simulink model "SPGF_FSK_0000_R2020b"  (R2020b)
settings: Solver=ode4  StartTime=0.0  StopTime=1.4  FixedStep=50e-6/50  RelTol=1e-3  EnableMultiTasking=on
undefined symbols (not defined in the file): D11, Delta
libraries: powerlib x2546, powerlib_meascontrol x183, simulink x24
(part 20 of 34)

== system SPGF_FSK_0000_R2020b/W31/DPL ==
  Ccs2/1 : powerlib/Elements/Series RLC Branch  LConnTagsString=__new0  RConnTagsString=__new0  BranchType=R  Resistance=-Rg_matrix(3,4)*2  Inductance=1e-3  SetiL0=off  InitialCurrent=0  Capacitance=Rg_matrix(3,4)*2  Setx0=off  InitialVoltage=0  Measurements=None
  Ccs2/3 : powerlib/Elements/Series RLC Branch  LConnTagsString=__new0  RConnTagsString=__new0  BranchType=R  Resistance=-Rg_matrix(3,4)*2  Inductance=1e-3  SetiL0=off  InitialCurrent=0  Capacitance=Rg_matrix(3,4)*2  Setx0=off  InitialVoltage=0  Measurements=None
  Ccs3/1 : powerlib/Elements/Series RLC Branch  LConnTagsString=__new0  RConnTagsString=__new0  BranchType=R  Resistance=-Rg_matrix(5,6)*2  Inductance=1e-3  SetiL0=off  InitialCurrent=0  Capacitance=-C_matrix(5,6)/2  Setx0=off  InitialVoltage=0  Measurements=None
  Ccs3/3 : powerlib/Elements/Series RLC Branch  LConnTagsString=__new0  RConnTagsString=__new0  BranchType=R  Resistance=-Rg_matrix(5,6)*2  Inductance=1e-3  SetiL0=off  InitialCurrent=0  Capacitance=-C_matrix(5,6)/2  Setx0=off  InitialVoltage=0  Measurements=None
  DPL : powerlib/Elements/Distributed Parameters Line  Phases=6  Length=LineLength  Frequency=Frequency  Resistance=R_matrix  Inductance=L_matrix  Capacitance=C_matrix  x1=[-3.15e-05 -1.16357054266887 0 -12.5014827360038 0 0 -9092.8182742179;-3.1e-05 -1.16390866949271 0 -12.505151651317 0 0 -9092.02733285201;-3.05e-05 -1.16424676759825 0 -12.5088202580778 0 0 -9091.23616714935;-3e-05 -1.16458483697715 0 -12.5124885561959 0 0 -9090.44477712942;-2.95e-05 -1.16492287762107 0 -12.5161565455808 0 0 -9089.65316281176;-2.9e-05 -1.16526088952168 0 -12.5198242261418 0 0 -9088.86132421589;-2.85e-05 -1.16559887267062 0 -12.5234915977886 0 0 -9088.06926136137;-2.8e-05 -1.16593682705957 0 -12.5271586604306 0 0 -9087.27697426772;-2.75e-05 -1.16627475268017 0 -12.5308254139773 0 0 -9086.4844629545;-2.7e-05 -1.1666126495241 0 -12.5344918583383 0 0 -9085.69172744126;-2.65e-05 -1.16695051758302 0 -12.5381579934231 0 0 -9084.89876774757;-2.6e-05 -1.16728835684859 0 -12.5418238191413 0 0 -9084.10558389299;-2.55e-05 -1.16762616731247 0 -12.5454893354024 0 0 -9083.31217589708;-2.5e-05 -1.16796394896633 0 -12.5491545421159 0 0 -9082.51854377943;-2.45e-05 -1.16830170180183 0 -12.5528194391915 0 0 -9081.72468755962;-2.4e-05 -1.16863942581065 0 -12.5564840265387 0 0 -9080.93060725724;-2.35e-05 -1.16897712098445 0 -12.560148304067 0 0 -9080.13630289187;-2.3e-05 -1.16931478731489 0 -12.5638122716861 0 0 -9079.34177448312;-2.25e-05 -1.16965242479364 0 -12.5674759293056 0 0 -9078.54702205059;-2.2e-05 -1.16999003341238 0 -12.571139276835 0 0 -9077.75204561389;-2.15e-05 -1.17032761316277 0 -12.574802314184 0 0 -9076.95684519264;-2.1e-05 -1.17066516403648 0 -12.5784650412621 0 0 -9076.16142080646;-2.05e-05 -1.17100268602519 0 -12.5821274579791 0 0 -9075.36577247497;-2e-05 -1.17134017912057 0 -12.5857895642446 0 0 -9074.56990021781;-1.95e-05 -1.17167764331428 0 -12.5894513599681 0 0 -9073.77380405461;-1.9e-05 -1.17201507859801 0 -12.5931128450594 0 0 -9072.97748400501;-1.85e-05 -1.17235248496343 0 -12.5967740194281 0 0 -9072.18094008867;-1.8e-05 -1.17268986240221 0 -12.6004348829838 0 0 -9071.38417232524;-1.75e-05 -1.17302721090602 0 -12.6040954356363 0 0 -9070.58718073438;-1.7e-05 -1.17336453046655 0 -12.6077556772951 0 0 -9069.78996533574;-1.65e-05 -1.17370182107547 0 -12.6114156078701 0 0 -9068.99252614901;-1.6e-05 -1.17403908272446 0 -12.6150752272709 0 0 -9068.19486319386;-1.55e-05 -1.17437631540519 0 -12.6187345354071 0 0 -9067.39697648997;-1.5e-05 -1.17471351910935 0 -12.6223935321886 0 0 -9066.59886605703;-1.45e-05 -1.17505069382862 0 -12.626052217525 0 0 -9065.80053191473;-1.4e-05 -1.17538783955467 0 -12.629710591326 0 0 -9065.00197408277;-1.35e-05 -1.17572495627919 0 -12.6333686535014 0 0 -9064.20319258085;-1.3e-05 -1.17606204399386 0 -12.637026403961 0 0 -9063.40418742868;-1.25e-05 -1.17639910269037 0 -12.6406838426144 0 0 -9062.60495864597;-1.2e-05 -1.17673613236039 0 -12.6443409693714 0 0 -9061.80550625245;-1.15e-05 -1.1770731329956 0 -12.6479977841419 0 0 -9061.00583026785;-1.1e-05 -1.17741010458771 0 -12.6516542868355 0 0 -9060.20593071188;-1.05e-05 -1.17774704712838 0 -12.655310477362 0 0 -9059.4058076043;-1e-05 -1.17808396060931 0 -12.6589663556313 0 0 -9058.60546096484;-9.5e-06 -1.17842084502218 0 -12.6626219215531 0 0 -9057.80489081324;-9e-06 -1.17875770035868 0 -12.6662771750372 0 0 -9057.00409716928;-8.5e-06 -1.17909452661051 0 -12.6699321159935 0 0 -9056.20308005269;-8e-06 -1.17943132376934 0 -12.6735867443317 0 0 -9055.40183948325;-7.5e-06 -1.17976809182687 0 -12.6772410599617 0 0 -9054.60037548072;-7e-06 -1.18010483077479 0 -12.6808950627934 0 0 -9053.79868806488;-6.5e-06 -1.18044154060479 0 -12.6845487527364 0 0 -9052.99677725552;-6e-06 -1.18077822130856 0 -12.6882021297008 0 0 -9052.19464307242;-5.5e-06 -1.1811148728778 5103.15019671596 -12.6918551935964 -2795.65081043936 4961.78174708621 -9051.39228553536;-5e-06 -1.1814514953042 5104.5723005975 -12.6955079443329 -2796.42987939011 4961.34178923313 -9050.58970466416;-4.5e-06 -1.18178808857945 5105.99427852876 -12.6991603818204 -2797.20887934172 4960.90170896385 -9049.7869004786;-4e-06 -1.18212465269524 5107.41613047466 -12.7028125059687 ...(+845 chars)]  x2=[-3.15e-05 -1.16269751442728 0 -12.461505127574 0 0 -9158.28571557594;-3.1e-05 -1.16304211630014 0 -12.4652625773679 0 0 -9157.49238310332;-3.05e-05 -1.16338668947608 0 -12.4690197195937 0 0 -9156.69882467864;-3e-05 -1.1637312339466 0 -12.4727765541588 0 0 -9155.90504032147;-2.95e-05 -1.16407574970321 0 -12.4765330809705 0 0 -9155.11103005139;-2.9e-05 -1.1644202367374 0 -12.480289299936 0 0 -9154.31679388801;-2.85e-05 -1.16476469504067 0 -12.4840452109628 0 0 -9153.52233185092;-2.8e-05 -1.16510912460452 0 -12.4878008139581 0 0 -9152.72764395971;-2.75e-05 -1.16545352542046 0 -12.4915561088292 0 0 -9151.932730234;-2.7e-05 -1.16579789747999 0 -12.4953110954836 0 0 -9151.1375906934;-2.65e-05 -1.1661422407746 0 -12.4990657738285 0 0 -9150.34222535754;-2.6e-05 -1.16648655529581 0 -12.5028201437714 0 0 -9149.54663424603;-2.55e-05 -1.16683084103512 0 -12.5065742052195 0 0 -9148.7508173785;-2.5e-05 -1.16717509798403 0 -12.5103279580803 0 0 -9147.9547747746;-2.45e-05 -1.16751932613405 0 -12.5140814022611 0 0 -9147.15850645397;-2.4e-05 -1.16786352547669 0 -12.5178345376693 0 0 -9146.36201243624;-2.35e-05 -1.16820769600344 0 -12.5215873642123 0 0 -9145.56529274108;-2.3e-05 -1.16855183770583 0 -12.5253398817976 0 0 -9144.76834738813;-2.25e-05 -1.16889595057536 0 -12.5290920903324 0 0 -9143.97117639708;-2.2e-05 -1.16924003460353 0 -12.5328439897244 0 0 -9143.17377978758;-2.15e-05 -1.16958408978187 0 -12.5365955798807 0 0 -9142.37615757931;-2.1e-05 -1.16992811610187 0 -12.540346860709 0 0 -9141.57830979194;-2.05e-05 -1.17027211355506 0 -12.5440978321167 0 0 -9140.78023644518;-2e-05 -1.17061608213293 0 -12.5478484940111 0 0 -9139.9819375587;-1.95e-05 -1.17096002182702 0 -12.5515988462998 0 0 -9139.18341315222;-1.9e-05 -1.17130393262882 0 -12.5553488888902 0 0 -9138.38466324541;-1.85e-05 -1.17164781452986 0 -12.5590986216898 0 0 -9137.58568785801;-1.8e-05 -1.17199166752164 0 -12.562848044606 0 0 -9136.78648700971;-1.75e-05 -1.17233549159569 0 -12.5665971575464 0 0 -9135.98706072025;-1.7e-05 -1.17267928674353 0 -12.5703459604184 0 0 -9135.18740900934;-1.65e-05 -1.17302305295666 0 -12.5740944531296 0 0 -9134.38753189672;-1.6e-05 -1.1733667902266 0 -12.5778426355874 0 0 -9133.58742940212;-1.55e-05 -1.17371049854489 0 -12.5815905076994 0 0 -9132.78710154528;-1.5e-05 -1.17405417790302 0 -12.5853380693731 0 0 -9131.98654834595;-1.45e-05 -1.17439782829253 0 -12.5890853205161 0 0 -9131.18576982389;-1.4e-05 -1.17474144970494 0 -12.5928322610358 0 0 -9130.38476599885;-1.35e-05 -1.17508504213176 0 -12.5965788908398 0 0 -9129.5835368906;-1.3e-05 -1.17542860556452 0 -12.6003252098357 0 0 -9128.7820825189;-1.25e-05 -1.17577213999474 0 -12.6040712179311 0 0 -9127.98040290353;-1.2e-05 -1.17611564541395 0 -12.6078169150334 0 0 -9127.17849806428;-1.15e-05 -1.17645912181367 0 -12.6115623010503 0 0 -9126.37636802092;-1.1e-05 -1.17680256918542 0 -12.6153073758894 0 0 -9125.57401279325;-1.05e-05 -1.17714598752073 0 -12.6190521394583 0 0 -9124.77143240107;-1e-05 -1.17748937681113 0 -12.6227965916646 0 0 -9123.96862686418;-9.5e-06 -1.17783273704815 0 -12.6265407324158 0 0 -9123.16559620239;-9e-06 -1.1781760682233 0 -12.6302845616196 0 0 -9122.3623404355;-8.5e-06 -1.17851937032813 0 -12.6340280791837 0 0 -9121.55885958335;-8e-06 -1.17886264335416 0 -12.6377712850155 0 0 -9120.75515366576;-7.5e-06 -1.17920588729292 0 -12.6415141790229 0 0 -9119.95122270256;-7e-06 -1.17954910213593 0 -12.6452567611135 0 0 -9119.14706671358;-6.5e-06 -1.17989228787475 0 -12.6489990311948 0 0 -9118.34268571866;-6e-06 -1.18023544450088 0 -12.6527409891746 0 0 -9117.53807973766;-5.5e-06 -1.18057857200588 5127.76906785034 -12.6564826349605 -2809.1377281476 4997.60028069833 -9116.73324879042;-5e-06 -1.18092167038126 5129.20187253766 -12.6602239684602 -2809.92265930412 4997.15896609033 -9115.9281928968;-4.5e-06 -1.18126473961857 5130.63455066699 -12.6639649895814 -2810.70752112858 4996.71752818238 -9115.12291207668;-4e-06 -1.18160777970934 5132.06710220299 -12.6677056982318 -2811.49231360161 ...(+828 chars)]  x3=[-3.15e-05 0.0167006451886816 0 -0.592002992330624 0 0 -460.167467556111;-3.1e-05 0.0166975880195327 0 -0.592580585093426 0 0 -460.166571304681;-3.05e-05 0.0166945304383873 0 -0.593158163234887 0 0 -460.165663699096;-3e-05 0.0166914724453209 0 -0.593735726740758 0 0 -460.164744739379;-2.95e-05 0.0166884140404089 0 -0.594313275596787 0 0 -460.163814425552;-2.9e-05 0.0166853552237268 0 -0.594890809788724 0 0 -460.162872757637;-2.85e-05 0.0166822959953501 0 -0.595468329302319 0 0 -460.161919735659;-2.8e-05 0.0166792363553542 0 -0.596045834123321 0 0 -460.160955359641;-2.75e-05 0.0166761763038147 0 -0.596623324237482 0 0 -460.159979629606;-2.7e-05 0.0166731158408069 0 -0.597200799630553 0 0 -460.158992545579;-2.65e-05 0.0166700549664066 0 -0.597778260288284 0 0 -460.157994107584;-2.6e-05 0.0166669936806891 0 -0.598355706196428 0 0 -460.156984315645;-2.55e-05 0.0166639319837301 0 -0.598933137340737 0 0 -460.155963169788;-2.5e-05 0.016660869875605 0 -0.599510553706963 0 0 -460.154930670038;-2.45e-05 0.0166578073563894 0 -0.600087955280859 0 0 -460.15388681642;-2.4e-05 0.0166547444261589 0 -0.600665342048179 0 0 -460.15283160896;-2.35e-05 0.0166516810849891 0 -0.601242713994675 0 0 -460.151765047684;-2.3e-05 0.0166486173329555 0 -0.601820071106101 0 0 -460.150687132618;-2.25e-05 0.0166455531701337 0 -0.602397413368213 0 0 -460.149597863789;-2.2e-05 0.0166424885965993 0 -0.602974740766764 0 0 -460.148497241224;-2.15e-05 0.0166394236124281 0 -0.603552053287511 0 0 -460.147385264949;-2.1e-05 0.0166363582176955 0 -0.604129350916207 0 0 -460.146261934994;-2.05e-05 0.0166332924124772 0 -0.604706633638609 0 0 -460.145127251384;-2e-05 0.0166302261968489 0 -0.605283901440472 0 0 -460.143981214148;-1.95e-05 0.0166271595708861 0 -0.605861154307554 0 0 -460.142823823315;-1.9e-05 0.0166240925346647 0 -0.606438392225612 0 0 -460.141655078912;-1.85e-05 0.0166210250882603 0 -0.607015615180401 0 0 -460.14047498097;-1.8e-05 0.0166179572317484 0 -0.607592823157681 0 0 -460.139283529516;-1.75e-05 0.0166148889652049 0 -0.608170016143209 0 0 -460.138080724581;-1.7e-05 0.0166118202887055 0 -0.608747194122744 0 0 -460.136866566193;-1.65e-05 0.0166087512023258 0 -0.609324357082043 0 0 -460.135641054384;-1.6e-05 0.0166056817061417 0 -0.609901505006866 0 0 -460.134404189182;-1.55e-05 0.0166026118002287 0 -0.610478637882974 0 0 -460.133155970619;-1.5e-05 0.0165995414846627 0 -0.611055755696124 0 0 -460.131896398726;-1.45e-05 0.0165964707595195 0 -0.611632858432078 0 0 -460.130625473533;-1.4e-05 0.0165933996248748 0 -0.612209946076596 0 0 -460.129343195073;-1.35e-05 0.0165903280808043 0 -0.612787018615439 0 0 -460.128049563375;-1.3e-05 0.0165872561273839 0 -0.613364076034369 0 0 -460.126744578474;-1.25e-05 0.0165841837646893 0 -0.613941118319147 0 0 -460.125428240399;-1.2e-05 0.0165811109927965 0 -0.614518145455535 0 0 -460.124100549185;-1.15e-05 0.0165780378117811 0 -0.615095157429295 0 0 -460.122761504864;-1.1e-05 0.016574964221719 0 -0.615672154226191 0 0 -460.121411107469;-1.05e-05 0.0165718902226861 0 -0.616249135831985 0 0 -460.120049357033;-1e-05 0.0165688158147581 0 -0.616826102232442 0 0 -460.11867625359;-9.5e-06 0.0165657409980111 0 -0.617403053413324 0 0 -460.117291797174;-9e-06 0.0165626657725207 0 -0.617979989360397 0 0 -460.115895987819;-8.5e-06 0.016559590138363 0 -0.618556910059424 0 0 -460.114488825558;-8e-06 0.0165565140956137 0 -0.619133815496172 0 0 -460.113070310429;-7.5e-06 0.0165534376443489 0 -0.619710705656405 0 0 -460.111640442464;-7e-06 0.0165503607846443 0 -0.62028758052589 0 0 -460.110199221699;-6.5e-06 0.016547283516576 0 -0.620864440090392 0 0 -460.10874664817;-6e-06 0.0165442058402198 0 -0.621441284335677 0 0 -460.107282721913;-5.5e-06 0.0165411277556516 -10.2033229098497 -0.622018113247514 -286.489948414025 588.173233513661 -460.105807442964;-5e-06 0.0165380492629475 -10.1348731635547 -0.622594926811669 -286.578402750177 588.127601544154 -460.10432081136;-4.5e-06 0.0165349703621835 -10.0664231671918 -0.62317172501391 ...(+981 chars)]  x4=[-3.15e-05 -0.0306851840034263 0 -1.23273715720339 0 0 174.215498589481;-3.1e-05 -0.0306862799089198 0 -1.23270367838231 0 0 174.239382593604;-3.05e-05 -0.0306873750572597 0 -1.23267016914548 0 0 174.263262298543;-3e-05 -0.0306884694484189 0 -1.23263662949374 0 0 174.287137703709;-2.95e-05 -0.0306895630823705 0 -1.23260305942791 0 0 174.311008808512;-2.9e-05 -0.0306906559590875 0 -1.23256945894881 0 0 174.334875612363;-2.85e-05 -0.0306917480785429 0 -1.23253582805729 0 0 174.358738114674;-2.8e-05 -0.0306928394407098 0 -1.23250216675416 0 0 174.382596314855;-2.75e-05 -0.0306939300455612 0 -1.23246847504026 0 0 174.406450212318;-2.7e-05 -0.0306950198930703 0 -1.23243475291642 0 0 174.430299806474;-2.65e-05 -0.0306961089832101 0 -1.23240100038347 0 0 174.454145096735;-2.6e-05 -0.0306971973159538 0 -1.23236721744224 0 0 174.477986082513;-2.55e-05 -0.0306982848912745 0 -1.23233340409358 0 0 174.501822763219;-2.5e-05 -0.0306993717091454 0 -1.2322995603383 0 0 174.525655138265;-2.45e-05 -0.0307004577695396 0 -1.23226568617725 0 0 174.549483207063;-2.4e-05 -0.0307015430724304 0 -1.23223178161127 0 0 174.573306969025;-2.35e-05 -0.0307026276177911 0 -1.23219784664118 0 0 174.597126423564;-2.3e-05 -0.0307037114055947 0 -1.23216388126783 0 0 174.620941570091;-2.25e-05 -0.0307047944358146 0 -1.23212988549206 0 0 174.644752408019;-2.2e-05 -0.0307058767084241 0 -1.2320958593147 0 0 174.668558936761;-2.15e-05 -0.0307069582233964 0 -1.23206180273659 0 0 174.692361155729;-2.1e-05 -0.030708038980705 0 -1.23202771575858 0 0 174.716159064335;-2.05e-05 -0.030709118980323 0 -1.2319935983815 0 0 174.739952661993;-2e-05 -0.0307101982222239 0 -1.23195945060619 0 0 174.763741948116;-1.95e-05 -0.030711276706381 0 -1.23192527243351 0 0 174.787526922116;-1.9e-05 -0.0307123544327678 0 -1.23189106386429 0 0 174.811307583406;-1.85e-05 -0.0307134314013576 0 -1.23185682489938 0 0 174.835083931401;-1.8e-05 -0.0307145076121238 0 -1.23182255553961 0 0 174.858855965513;-1.75e-05 -0.03071558306504 0 -1.23178825578585 0 0 174.882623685155;-1.7e-05 -0.0307166577600795 0 -1.23175392563892 0 0 174.906387089742;-1.65e-05 -0.0307177316972158 0 -1.23171956509969 0 0 174.930146178687;-1.6e-05 -0.0307188048764226 0 -1.23168517416899 0 0 174.953900951403;-1.55e-05 -0.0307198772976731 0 -1.23165075284768 0 0 174.977651407305;-1.5e-05 -0.0307209489609411 0 -1.23161630113661 0 0 175.001397545806;-1.45e-05 -0.0307220198662001 0 -1.23158181903662 0 0 175.025139366321;-1.4e-05 -0.0307230900134236 0 -1.23154730654857 0 0 175.048876868263;-1.35e-05 -0.0307241594025853 0 -1.23151276367331 0 0 175.072610051048;-1.3e-05 -0.0307252280336587 0 -1.23147819041169 0 0 175.09633891409;-1.25e-05 -0.0307262959066175 0 -1.23144358676456 0 0 175.120063456802;-1.2e-05 -0.0307273630214353 0 -1.23140895273278 0 0 175.1437836786;-1.15e-05 -0.0307284293780858 0 -1.2313742883172 0 0 175.167499578898;-1.1e-05 -0.0307294949765428 0 -1.23133959351868 0 0 175.191211157112;-1.05e-05 -0.0307305598167798 0 -1.23130486833807 0 0 175.214918412655;-1e-05 -0.0307316238987707 0 -1.23127011277623 0 0 175.238621344944;-9.5e-06 -0.0307326872224891 0 -1.23123532683402 0 0 175.262319953393;-9e-06 -0.0307337497879089 0 -1.2312005105123 0 0 175.286014237418;-8.5e-06 -0.0307348115950038 0 -1.23116566381192 0 0 175.309704196434;-8e-06 -0.0307358726437477 0 -1.23113078673375 0 0 175.333389829856;-7.5e-06 -0.0307369329341142 0 -1.23109587927864 0 0 175.3570711371;-7e-06 -0.0307379924660774 0 -1.23106094144746 0 0 175.380748117582;-6.5e-06 -0.030739051239611 0 -1.23102597324106 0 0 175.404420770717;-6e-06 -0.0307401092546889 0 -1.23099097466032 0 0 175.428089095922;-5.5e-06 -0.030741166511285 146.635682578115 -1.2309559457061 -218.849985399863 372.665529908053 175.451753092612;-5e-06 -0.0307422230093732 146.605378031747 -1.23092088637925 -218.902824837774 372.626298068453 175.475412760204;-4.5e-06 -0.0307432787489275 146.575069868035 -1.23088579668065 -218.955658874474 372.587057034668 175.499068098113;-4e-06 ...(+905 chars)]  x5=3.11781574821658e-05  V1=ones(3,3)  V2=ones(3,3)  I1=ones(3,3)  I2=ones(3,3)  nHarmo=1  Measurements=None  Decoupling=off  VsMag0=0  VrMag0=0  VsAngle0=0  VrAngle0=0  IsMag0=0  IrMag0=0  IsAngle0=0  IrAngle0=0
  Ground{1..4} (4 alike) : powerlib/Elements/Ground  LConnTagsString=a
  Rcs*1 : powerlib/Elements/Series RLC Branch  LConnTagsString=__new0  RConnTagsString=__new0  BranchType=R  Resistance=-Rg_matrix(1,2)*2  Inductance=1e-3  SetiL0=off  InitialCurrent=0  Capacitance=Rg_matrix(1,2)*2  Setx0=off  InitialVoltage=0  Measurements=None
  Rcs*2 : powerlib/Elements/Series RLC Branch  LConnTagsString=__new0  RConnTagsString=__new0  BranchType=R  Resistance=-Rg_matrix(1,2)*2  Inductance=1e-3  SetiL0=off  InitialCurrent=0  Capacitance=Rg_matrix(1,2)*2  Setx0=off  InitialVoltage=0  Measurements=None
  Rgsg1/1 : powerlib/Elements/Series RLC Branch  LConnTagsString=__new0  RConnTagsString=__new0  BranchType=R  Resistance=(Rg_matrix(4,4)+Rg_matrix(3,4))*2  Inductance=1e-3  SetiL0=off  InitialCurrent=0  Capacitance=Rg_matrix(1,2)*2  Setx0=off  InitialVoltage=0  Measurements=None
  Rgsg1/2 : powerlib/Elements/Series RLC Branch  LConnTagsString=__new0  RConnTagsString=__new0  BranchType=R  Resistance=(Rg_matrix(2,2)+Rg_matrix(1,2))*2  Inductance=1e-3  SetiL0=off  InitialCurrent=0  Capacitance=Rg_matrix(1,2)*2  Setx0=off  InitialVoltage=0  Measurements=None
  Rgsg1/3 : powerlib/Elements/Series RLC Branch  LConnTagsString=__new0  RConnTagsString=__new0  BranchType=R  Resistance=(Rg_matrix(4,4)+Rg_matrix(3,4))*2  Inductance=1e-3  SetiL0=off  InitialCurrent=0  Capacitance=Rg_matrix(1,2)*2  Setx0=off  InitialVoltage=0  Measurements=None
  Rgsg1/4 : powerlib/Elements/Series RLC Branch  LConnTagsString=__new0  RConnTagsString=__new0  BranchType=R  Resistance=(Rg_matrix(2,2)+Rg_matrix(1,2))*2  Inductance=1e-3  SetiL0=off  InitialCurrent=0  Capacitance=Rg_matrix(1,2)*2  Setx0=off  InitialVoltage=0  Measurements=None
  Rsg*1 : powerlib/Elements/Series RLC Branch  LConnTagsString=__new0  RConnTagsString=__new0  BranchType=R  Resistance=(Rg_matrix(6,6)+Rg_matrix(5,6))*2  Inductance=1e-3  SetiL0=off  InitialCurrent=0  Capacitance=Rg_matrix(1,2)*2  Setx0=off  InitialVoltage=0  Measurements=None
  Rsg*2 : powerlib/Elements/Series RLC Branch  LConnTagsString=__new0  RConnTagsString=__new0  BranchType=R  Resistance=(Rg_matrix(6,6)+Rg_matrix(5,6))*2  Inductance=1e-3  SetiL0=off  InitialCurrent=0  Capacitance=Rg_matrix(1,2)*2  Setx0=off  InitialVoltage=0  Measurements=None
  A : PMIOPort  Side=Left
  B : PMIOPort  Port=2  Side=Left
  C : PMIOPort  Port=3  Side=Left
  a : PMIOPort  Port=4  Side=Right
  b : PMIOPort  Port=5  Side=Right
  c : PMIOPort  Port=6  Side=Right
  connections:
  c/RConn1 -- Ccs3/1/RConn1 -- DPL/RConn5
  b/RConn1 -- Ccs2/1/RConn1 -- DPL/RConn3
  a/RConn1 -- DPL/RConn1 -- Rcs*1/RConn1
  Ground4/LConn1 -- DPL/RConn6 -- Ccs3/1/LConn1 -- Rsg*1/LConn1 -- Rcs*1/LConn1 -- Rgsg1/4/LConn1 -- DPL/RConn2 -- DPL/RConn4 -- Ccs2/1/LConn1 -- Rgsg1/3/LConn1
  Ground1/LConn1 -- Rgsg1/4/RConn1 -- Rsg*1/RConn1 -- Rgsg1/3/RConn1
  Ground3/LConn1 -- Ccs3/3/LConn1 -- Rsg*2/LConn1 -- DPL/LConn6 -- Rgsg1/1/LConn1 -- Ccs2/3/LConn1 -- DPL/LConn4 -- Rgsg1/2/LConn1 -- Rcs*2/LConn1 -- DPL/LConn2
  Ground2/LConn1 -- Rgsg1/1/RConn1 -- Rsg*2/RConn1 -- Rgsg1/2/RConn1
  Ccs3/3/RConn1 -- DPL/LConn5 -- C/RConn1
  Ccs2/3/RConn1 -- DPL/LConn3 -- B/RConn1
  Rcs*2/RConn1 -- DPL/LConn1 -- A/RConn1

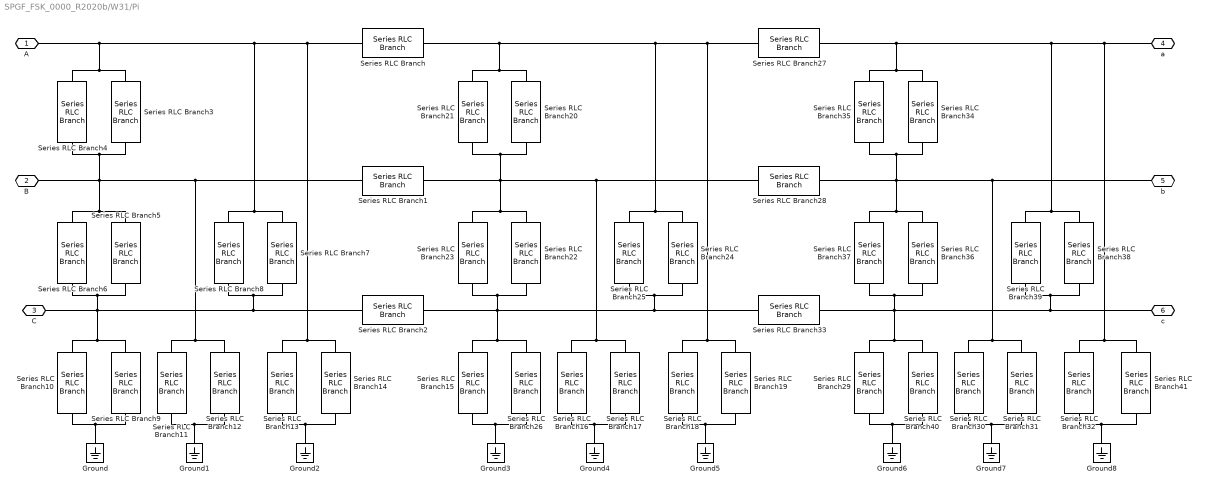
== system SPGF_FSK_0000_R2020b/W31/Pi ==
  Ground{,1..8} (9 alike) : powerlib/Elements/Ground  LConnTagsString=a
  Series RLC Branch{,1..2,27..28,33} (6 alike) : powerlib/Elements/Series RLC Branch  LConnTagsString=__new0  RConnTagsString=__new0  BranchType=RL  Resistance=R/2  Inductance=L/2  SetiL0=off  InitialCurrent=0  Capacitance=1e-6  Setx0=off  InitialVoltage=0  Measurements=None
  Series RLC Branch{10..11,13,29..30,32} (6 alike) : powerlib/Elements/Series RLC Branch  LConnTagsString=__new0  RConnTagsString=__new0  BranchType=R  Resistance=Rfg*4  Inductance=L/2  SetiL0=off  InitialCurrent=0  Capacitance=1e-6  Setx0=off  InitialVoltage=0  Measurements=None
  Series RLC Branch{9,12,14,31,40..41} (6 alike) : powerlib/Elements/Series RLC Branch  LConnTagsString=__new0  RConnTagsString=__new0  BranchType=C  Resistance=R/2  Inductance=L/2  SetiL0=off  InitialCurrent=0  Capacitance=Cfg*0.25  Setx0=off  InitialVoltage=0  Measurements=None
  Series RLC Branch15 : powerlib/Elements/Series RLC Branch  LConnTagsString=__new0  RConnTagsString=__new0  BranchType=R  Resistance=Rfg*2  Inductance=L/2  SetiL0=off  InitialCurrent=0  Capacitance=1e-6  Setx0=off  InitialVoltage=0  Measurements=None
  Series RLC Branch16 : powerlib/Elements/Series RLC Branch  LConnTagsString=__new0  RConnTagsString=__new0  BranchType=R  Resistance=Rfg*2  Inductance=L/2  SetiL0=off  InitialCurrent=0  Capacitance=1e-6  Setx0=off  InitialVoltage=0  Measurements=None
  Series RLC Branch17 : powerlib/Elements/Series RLC Branch  LConnTagsString=__new0  RConnTagsString=__new0  BranchType=C  Resistance=R/2  Inductance=L/2  SetiL0=off  InitialCurrent=0  Capacitance=Cfg*0.5  Setx0=off  InitialVoltage=0  Measurements=None
  Series RLC Branch18 : powerlib/Elements/Series RLC Branch  LConnTagsString=__new0  RConnTagsString=__new0  BranchType=R  Resistance=Rfg*2  Inductance=L/2  SetiL0=off  InitialCurrent=0  Capacitance=1e-6  Setx0=off  InitialVoltage=0  Measurements=None
  Series RLC Branch19 : powerlib/Elements/Series RLC Branch  LConnTagsString=__new0  RConnTagsString=__new0  BranchType=C  Resistance=R/2  Inductance=L/2  SetiL0=off  InitialCurrent=0  Capacitance=Cfg*0.5  Setx0=off  InitialVoltage=0  Measurements=None
  Series RLC Branch20 : powerlib/Elements/Series RLC Branch  LConnTagsString=__new0  RConnTagsString=__new0  BranchType=C  Resistance=R/2  Inductance=L/2  SetiL0=off  InitialCurrent=0  Capacitance=Cmf*0.5  Setx0=off  InitialVoltage=0  Measurements=None
  Series RLC Branch21 : powerlib/Elements/Series RLC Branch  LConnTagsString=__new0  RConnTagsString=__new0  BranchType=R  Resistance=Rmf*2  Inductance=L/2  SetiL0=off  InitialCurrent=0  Capacitance=1e-6  Setx0=off  InitialVoltage=0  Measurements=None
  Series RLC Branch22 : powerlib/Elements/Series RLC Branch  LConnTagsString=__new0  RConnTagsString=__new0  BranchType=C  Resistance=R/2  Inductance=L/2  SetiL0=off  InitialCurrent=0  Capacitance=Cmf*0.5  Setx0=off  InitialVoltage=0  Measurements=None
  Series RLC Branch23 : powerlib/Elements/Series RLC Branch  LConnTagsString=__new0  RConnTagsString=__new0  BranchType=R  Resistance=Rmf*2  Inductance=L/2  SetiL0=off  InitialCurrent=0  Capacitance=1e-6  Setx0=off  InitialVoltage=0  Measurements=None
  Series RLC Branch24 : powerlib/Elements/Series RLC Branch  LConnTagsString=__new0  RConnTagsString=__new0  BranchType=C  Resistance=R/2  Inductance=L/2  SetiL0=off  InitialCurrent=0  Capacitance=Cmf*0.5  Setx0=off  InitialVoltage=0  Measurements=None
  Series RLC Branch25 : powerlib/Elements/Series RLC Branch  LConnTagsString=__new0  RConnTagsString=__new0  BranchType=R  Resistance=Rmf*2  Inductance=L/2  SetiL0=off  InitialCurrent=0  Capacitance=1e-6  Setx0=off  InitialVoltage=0  Measurements=None
  Series RLC Branch26 : powerlib/Elements/Series RLC Branch  LConnTagsString=__new0  RConnTagsString=__new0  BranchType=C  Resistance=R/2  Inductance=L/2  SetiL0=off  InitialCurrent=0  Capacitance=Cfg*0.5  Setx0=off  InitialVoltage=0  Measurements=None
  Series RLC Branch{3,5,7,34,36,38} (6 alike) : powerlib/Elements/Series RLC Branch  LConnTagsString=__new0  RConnTagsString=__new0  BranchType=C  Resistance=R/2  Inductance=L/2  SetiL0=off  InitialCurrent=0  Capacitance=Cmf*0.25  Setx0=off  InitialVoltage=0  Measurements=None
  Series RLC Branch{4,6,8,35,37,39} (6 alike) : powerlib/Elements/Series RLC Branch  LConnTagsString=__new0  RConnTagsString=__new0  BranchType=R  Resistance=Rmf*4  Inductance=L/2  SetiL0=off  InitialCurrent=0  Capacitance=1e-6  Setx0=off  InitialVoltage=0  Measurements=None
  A : PMIOPort  Side=Left
  B : PMIOPort  Port=2  Side=Left
  C : PMIOPort  Port=3  Side=Left
  a : PMIOPort  Port=4  Side=Right
  b : PMIOPort  Port=5  Side=Right
  c : PMIOPort  Port=6  Side=Right
  connections:
  Ground8/LConn1 -- Series RLC Branch41/RConn1 -- Series RLC Branch32/RConn1
  Ground7/LConn1 -- Series RLC Branch30/RConn1 -- Series RLC Branch31/RConn1
  Ground6/LConn1 -- Series RLC Branch40/RConn1 -- Series RLC Branch29/RConn1
  Series RLC Branch40/LConn1 -- Series RLC Branch33/RConn1 -- Series RLC Branch38/RConn1 -- Series RLC Branch39/RConn1 -- c/RConn1 -- Series RLC Branch37/RConn1 -- Series RLC Branch36/RConn1 -- Series RLC Branch29/LConn1
  Series RLC Branch35/LConn1 -- Series RLC Branch27/RConn1 -- Series RLC Branch39/LConn1 -- Series RLC Branch38/LConn1 -- Series RLC Branch32/LConn1 -- Series RLC Branch41/LConn1 -- a/RConn1 -- Series RLC Branch34/LConn1
  Series RLC Branch30/LConn1 -- Series RLC Branch28/RConn1 -- Series RLC Branch37/LConn1 -- Series RLC Branch36/LConn1 -- Series RLC Branch34/RConn1 -- Series RLC Branch35/RConn1 -- b/RConn1 -- Series RLC Branch31/LConn1
  Series RLC Branch19/RConn1 -- Series RLC Branch18/RConn1 -- Ground5/LConn1
  Series RLC Branch16/RConn1 -- Series RLC Branch17/RConn1 -- Ground4/LConn1
  Ground3/LConn1 -- Series RLC Branch15/RConn1 -- Series RLC Branch26/RConn1
  Series RLC Branch23/RConn1 -- Series RLC Branch22/RConn1 -- Series RLC Branch24/RConn1 -- Series RLC Branch25/RConn1 -- Series RLC Branch33/LConn1 -- Series RLC Branch2/RConn1 -- Series RLC Branch15/LConn1 -- Series RLC Branch26/LConn1
  Series RLC Branch25/LConn1 -- Series RLC Branch24/LConn1 -- Series RLC Branch18/LConn1 -- Series RLC Branch19/LConn1 -- Series RLC Branch27/LConn1 -- Series RLC Branch/RConn1 -- Series RLC Branch20/LConn1 -- Series RLC Branch21/LConn1
  Series RLC Branch21/RConn1 -- Series RLC Branch20/RConn1 -- Series RLC Branch22/LConn1 -- Series RLC Branch23/LConn1 -- Series RLC Branch1/RConn1 -- Series RLC Branch28/LConn1 -- Series RLC Branch16/LConn1 -- Series RLC Branch17/LConn1
  Ground2/LConn1 -- Series RLC Branch14/RConn1 -- Series RLC Branch13/RConn1
  Ground1/LConn1 -- Series RLC Branch11/RConn1 -- Series RLC Branch12/RConn1
  Series RLC Branch10/RConn1 -- Ground/LConn1 -- Series RLC Branch9/RConn1
  Series RLC Branch10/LConn1 -- Series RLC Branch6/RConn1 -- Series RLC Branch5/RConn1 -- C/RConn1 -- Series RLC Branch7/RConn1 -- Series RLC Branch8/RConn1 -- Series RLC Branch2/LConn1 -- Series RLC Branch9/LConn1
  Series RLC Branch14/LConn1 -- Series RLC Branch/LConn1 -- Series RLC Branch8/LConn1 -- Series RLC Branch7/LConn1 -- Series RLC Branch3/LConn1 -- Series RLC Branch4/LConn1 -- A/RConn1 -- Series RLC Branch13/LConn1
  Series RLC Branch1/LConn1 -- Series RLC Branch3/RConn1 -- Series RLC Branch4/RConn1 -- B/RConn1 -- Series RLC Branch6/LConn1 -- Series RLC Branch5/LConn1 -- Series RLC Branch11/LConn1 -- Series RLC Branch12/LConn1

== system SPGF_FSK_0000_R2020b/W31/Q ==
  breaker : Subsystem  Commented=on  mask{SwitchA=on, SwitchB=on, SwitchC=on, InitialStatus=[0 0 0], BreakerResistance=0.0001, SnubberResistance=1e6, SnubberCapacitance=inf, TransitionTimes=[0.2], ShiftTimes=[0 0.02 0.025]}
      mask prompts: SwitchA "Switching of phase A"; SwitchB "Switching of phase B"; SwitchC "Switching of phase C"; InitialStatus "Initial status of phase breaker [A, B, C]"; BreakerResistance "Breaker resistance Ron (ohms) :"; SnubberResistance "Snubbers resistance Rp (ohms) :"; SnubberCapacitance "Snubbers capacitance Cp (F) :"; TransitionTimes "Transition times (s) :"; ShiftTimes "Time differences for switch [tA, tB, tC] (s) :"
      mask init: same as SPGF_FSK_0000_R2020b/Feed/Q/breaker
      mask Display:
      | % port_label('input',1,'Iabc');
      | 
      | port_label('lconn',1,'A');
      | port_label('lconn',2,'B');
      | port_label('lconn',3,'C');
      | 
      | port_label('rconn',1,'a');
      | port_label('rconn',2,'b');
      | port_label('rconn',3,'c');
      | 
      | disp('   Q    ');
  meas : Subsystem
  shunt : Subsystem
  A : PMIOPort  Side=Right
  B : PMIOPort  Port=2  Side=Right
  C : PMIOPort  Port=3  Side=Right
  a : PMIOPort  Port=4  Side=Left
  b : PMIOPort  Port=5  Side=Left
  c : PMIOPort  Port=6  Side=Left
  connections:
  shunt/LConn3 -- breaker/LConn3 -- C/RConn1
  shunt/LConn2 -- breaker/LConn2 -- B/RConn1
  A/RConn1 -- breaker/LConn1 -- shunt/LConn1
  meas/RConn1 -- a/RConn1
  meas/RConn2 -- b/RConn1
  meas/RConn3 -- c/RConn1
  meas/LConn3 -- breaker/RConn3 -- shunt/RConn3
  meas/LConn2 -- breaker/RConn2 -- shunt/RConn2
  meas/LConn1 -- breaker/RConn1 -- shunt/RConn1

== system SPGF_FSK_0000_R2020b/W31/concentrated ==
  Ccs/1 : powerlib/Elements/Series RLC Branch  LConnTagsString=__new0  RConnTagsString=__new0  BranchType=C  Resistance=190  Inductance=1e-3  SetiL0=off  InitialCurrent=0  Capacitance=-C_matrix(1,2)/2  Setx0=off  InitialVoltage=0  Measurements=None
  Ccs/2 : powerlib/Elements/Series RLC Branch  LConnTagsString=__new0  RConnTagsString=__new0  BranchType=C  Resistance=190  Inductance=1e-3  SetiL0=off  InitialCurrent=0  Capacitance=-C_matrix(1,2)/2  Setx0=off  InitialVoltage=0  Measurements=None
  Ccs2/1 : powerlib/Elements/Series RLC Branch  LConnTagsString=__new0  RConnTagsString=__new0  BranchType=C  Resistance=190  Inductance=1e-3  SetiL0=off  InitialCurrent=0  Capacitance=-C_matrix(3,4)/2  Setx0=off  InitialVoltage=0  Measurements=None
  Ccs2/2 : powerlib/Elements/Series RLC Branch  LConnTagsString=__new0  RConnTagsString=__new0  BranchType=C  Resistance=190  Inductance=1e-3  SetiL0=off  InitialCurrent=0  Capacitance=-C_matrix(3,4)/2  Setx0=off  InitialVoltage=0  Measurements=None
  Ccs2/3 : powerlib/Elements/Series RLC Branch  LConnTagsString=__new0  RConnTagsString=__new0  BranchType=R  Resistance=-Rg_matrix(3,4)*2  Inductance=1e-3  SetiL0=off  InitialCurrent=0  Capacitance=Rg_matrix(3,4)*2  Setx0=off  InitialVoltage=0  Measurements=None
  Ccs2/4 : powerlib/Elements/Series RLC Branch  LConnTagsString=__new0  RConnTagsString=__new0  BranchType=R  Resistance=-Rg_matrix(3,4)*2  Inductance=1e-3  SetiL0=off  InitialCurrent=0  Capacitance=Rg_matrix(3,4)*2  Setx0=off  InitialVoltage=0  Measurements=None
  Ccs3/1 : powerlib/Elements/Series RLC Branch  LConnTagsString=__new0  RConnTagsString=__new0  BranchType=C  Resistance=190  Inductance=1e-3  SetiL0=off  InitialCurrent=0  Capacitance=-C_matrix(5,6)/2  Setx0=off  InitialVoltage=0  Measurements=None
  Ccs3/2 : powerlib/Elements/Series RLC Branch  LConnTagsString=__new0  RConnTagsString=__new0  BranchType=C  Resistance=190  Inductance=1e-3  SetiL0=off  InitialCurrent=0  Capacitance=-C_matrix(5,6)/2  Setx0=off  InitialVoltage=0  Measurements=None
  Ccs3/3 : powerlib/Elements/Series RLC Branch  LConnTagsString=__new0  RConnTagsString=__new0  BranchType=R  Resistance=-Rg_matrix(5,6)*2  Inductance=1e-3  SetiL0=off  InitialCurrent=0  Capacitance=-C_matrix(5,6)/2  Setx0=off  InitialVoltage=0  Measurements=None
  Ccs3/4 : powerlib/Elements/Series RLC Branch  LConnTagsString=__new0  RConnTagsString=__new0  BranchType=R  Resistance=-Rg_matrix(5,6)*2  Inductance=1e-3  SetiL0=off  InitialCurrent=0  Capacitance=-C_matrix(5,6)/2  Setx0=off  InitialVoltage=0  Measurements=None
  Csg/2 : powerlib/Elements/Series RLC Branch  LConnTagsString=__new0  RConnTagsString=__new0  BranchType=C  Resistance=190  Inductance=1e-3  SetiL0=off  InitialCurrent=0  Capacitance=( C_matrix(1,2) + C_matrix(2,2) )/2  Setx0=off  InitialVoltage=0  Measurements=None
  Csg1/1 : powerlib/Elements/Series RLC Branch  LConnTagsString=__new0  RConnTagsString=__new0  BranchType=C  Resistance=190  Inductance=1e-3  SetiL0=off  InitialCurrent=0  Capacitance=( C_matrix(1,2) + C_matrix(2,2) )/2  Setx0=off  InitialVoltage=0  Measurements=None
  Csg2/1 : powerlib/Elements/Series RLC Branch  LConnTagsString=__new0  RConnTagsString=__new0  BranchType=C  Resistance=190  Inductance=1e-3  SetiL0=off  InitialCurrent=0  Capacitance=( C_matrix(3,4) + C_matrix(4,4) )/2  Setx0=off  InitialVoltage=0  Measurements=None
  Csg2/2 : powerlib/Elements/Series RLC Branch  LConnTagsString=__new0  RConnTagsString=__new0  BranchType=C  Resistance=190  Inductance=1e-3  SetiL0=off  InitialCurrent=0  Capacitance=( C_matrix(3,4) + C_matrix(4,4) )/2  Setx0=off  InitialVoltage=0  Measurements=None
  Csg3/1 : powerlib/Elements/Series RLC Branch  LConnTagsString=__new0  RConnTagsString=__new0  BranchType=C  Resistance=190  Inductance=1e-3  SetiL0=off  InitialCurrent=0  Capacitance=( C_matrix(5,6) + C_matrix(6,6) ) /2  Setx0=off  InitialVoltage=0  Measurements=None
  Csg3/2 : powerlib/Elements/Series RLC Branch  LConnTagsString=__new0  RConnTagsString=__new0  BranchType=C  Resistance=190  Inductance=1e-3  SetiL0=off  InitialCurrent=0  Capacitance=( C_matrix(5,6) + C_matrix(6,6) ) /2  Setx0=off  InitialVoltage=0  Measurements=None
  Ground{1..4} (4 alike) : powerlib/Elements/Ground  LConnTagsString=a
  RL : powerlib/Elements/Mutual Inductance  LConnTagsString=a|b|c|L4|L5|L6  RConnTagsString=A|B|C|R4|R5|R6  TypeOfMutual=Generalized mutual inductance  NumberOfWindings=6  SelfImpedance1=[1.1 1.1e-03]  SelfImpedance2=[ 1.1 1.1e-03]  ThreeWindings=on  SelfImpedance3=[ 1.1 1.1e-03]  MutualImpedance=[1.0 1.0e-03]  InductanceMatrix=L_matrix  ResistanceMatrix=R_matrix  Measurements=None
      settings: AttributesFormatString=\n
  Rcs*2 : powerlib/Elements/Series RLC Branch  LConnTagsString=__new0  RConnTagsString=__new0  BranchType=R  Resistance=-Rg_matrix(1,2)*2  Inductance=1e-3  SetiL0=off  InitialCurrent=0  Capacitance=Rg_matrix(1,2)*2  Setx0=off  InitialVoltage=0  Measurements=None
  Rgcs1/1 : powerlib/Elements/Series RLC Branch  LConnTagsString=__new0  RConnTagsString=__new0  BranchType=R  Resistance=-Rg_matrix(1,2)*2  Inductance=1e-3  SetiL0=off  InitialCurrent=0  Capacitance=Rg_matrix(1,2)*2  Setx0=off  InitialVoltage=0  Measurements=None
  Rgsg1/1 : powerlib/Elements/Series RLC Branch  LConnTagsString=__new0  RConnTagsString=__new0  BranchType=R  Resistance=(Rg_matrix(4,4)+Rg_matrix(3,4))*2  Inductance=1e-3  SetiL0=off  InitialCurrent=0  Capacitance=Rg_matrix(1,2)*2  Setx0=off  InitialVoltage=0  Measurements=None
  Rgsg1/2 : powerlib/Elements/Series RLC Branch  LConnTagsString=__new0  RConnTagsString=__new0  BranchType=R  Resistance=(Rg_matrix(2,2)+Rg_matrix(1,2))*2  Inductance=1e-3  SetiL0=off  InitialCurrent=0  Capacitance=Rg_matrix(1,2)*2  Setx0=off  InitialVoltage=0  Measurements=None
  Rgsg1/3 : powerlib/Elements/Series RLC Branch  LConnTagsString=__new0  RConnTagsString=__new0  BranchType=R  Resistance=(Rg_matrix(4,4)+Rg_matrix(3,4))*2  Inductance=1e-3  SetiL0=off  InitialCurrent=0  Capacitance=Rg_matrix(1,2)*2  Setx0=off  InitialVoltage=0  Measurements=None
  Rgsg1/4 : powerlib/Elements/Series RLC Branch  LConnTagsString=__new0  RConnTagsString=__new0  BranchType=R  Resistance=(Rg_matrix(2,2)+Rg_matrix(1,2))*2  Inductance=1e-3  SetiL0=off  InitialCurrent=0  Capacitance=Rg_matrix(1,2)*2  Setx0=off  InitialVoltage=0  Measurements=None
  Rsg*2 : powerlib/Elements/Series RLC Branch  LConnTagsString=__new0  RConnTagsString=__new0  BranchType=R  Resistance=(Rg_matrix(6,6)+Rg_matrix(5,6))*2  Inductance=1e-3  SetiL0=off  InitialCurrent=0  Capacitance=Rg_matrix(1,2)*2  Setx0=off  InitialVoltage=0  Measurements=None
  Rsg1/1 : powerlib/Elements/Series RLC Branch  LConnTagsString=__new0  RConnTagsString=__new0  BranchType=R  Resistance=(Rg_matrix(6,6)+Rg_matrix(5,6))*2  Inductance=1e-3  SetiL0=off  InitialCurrent=0  Capacitance=Rg_matrix(1,2)*2  Setx0=off  InitialVoltage=0  Measurements=None
  A : PMIOPort  Side=Left
  B : PMIOPort  Port=2  Side=Left
  C : PMIOPort  Port=3  Side=Left
  a : PMIOPort  Port=4  Side=Right
  b : PMIOPort  Port=5  Side=Right
  c : PMIOPort  Port=6  Side=Right
  connections:
  Ccs3/3/RConn1 -- RL/LConn5 -- C/RConn1 -- Ccs3/2/RConn1
  Ccs2/2/RConn1 -- Ccs2/3/RConn1 -- B/RConn1 -- RL/LConn3
  Ccs/2/RConn1 -- Rcs*2/RConn1 -- A/RConn1 -- RL/LConn1
  Ccs3/4/RConn1 -- RL/RConn5 -- c/RConn1 -- Ccs3/1/RConn1
  Ccs2/1/RConn1 -- Ccs2/4/RConn1 -- RL/RConn3 -- b/RConn1
  Ccs/1/RConn1 -- Rgcs1/1/RConn1 -- RL/RConn1 -- a/RConn1
  Csg/2/RConn1 -- Ground1/LConn1 -- Csg2/2/RConn1 -- Csg3/2/RConn1 -- Rgsg1/2/RConn1 -- Rgsg1/1/RConn1 -- Rsg*2/RConn1
  Csg3/1/LConn1 -- Ccs3/4/LConn1 -- Rsg1/1/LConn1 -- Ccs3/1/LConn1 -- RL/RConn6 -- Ground4/LConn1 -- RL/RConn2 -- Ccs/1/LConn1 -- Csg1/1/LConn1 -- Rgcs1/1/LConn1 -- Rgsg1/4/LConn1 -- RL/RConn4 -- Ccs2/1/LConn1 -- Csg2/1/LConn1 -- Ccs2/4/LConn1 -- Rgsg1/3/LConn1
  Csg1/1/RConn1 -- Ground2/LConn1 -- Csg2/1/RConn1 -- Csg3/1/RConn1 -- Rgsg1/4/RConn1 -- Rgsg1/3/RConn1 -- Rsg1/1/RConn1
  Ccs3/2/LConn1 -- Ccs3/3/LConn1 -- Csg3/2/LConn1 -- Rsg*2/LConn1 -- Ccs2/2/LConn1 -- Ccs2/3/LConn1 -- Csg2/2/LConn1 -- Rgsg1/1/LConn1 -- RL/LConn4 -- RL/LConn2 -- Ccs/2/LConn1 -- Rcs*2/LConn1 -- Csg/2/LConn1 -- Rgsg1/2/LConn1 -- Ground3/LConn1 -- RL/LConn6
